simulink model "decimation"  (R2013b)
settings: Solver=ode45  StartTime=0.0  StopTime=10.0  RelTol=1e-3
undefined symbols (not defined in the file): xlfda_numerator
libraries: xbsIndex_r4 x1962, xps_library x2, casper_library_misc x1
(part 1 of 19)
settings Model: Creator=root  LastModifiedBy=root

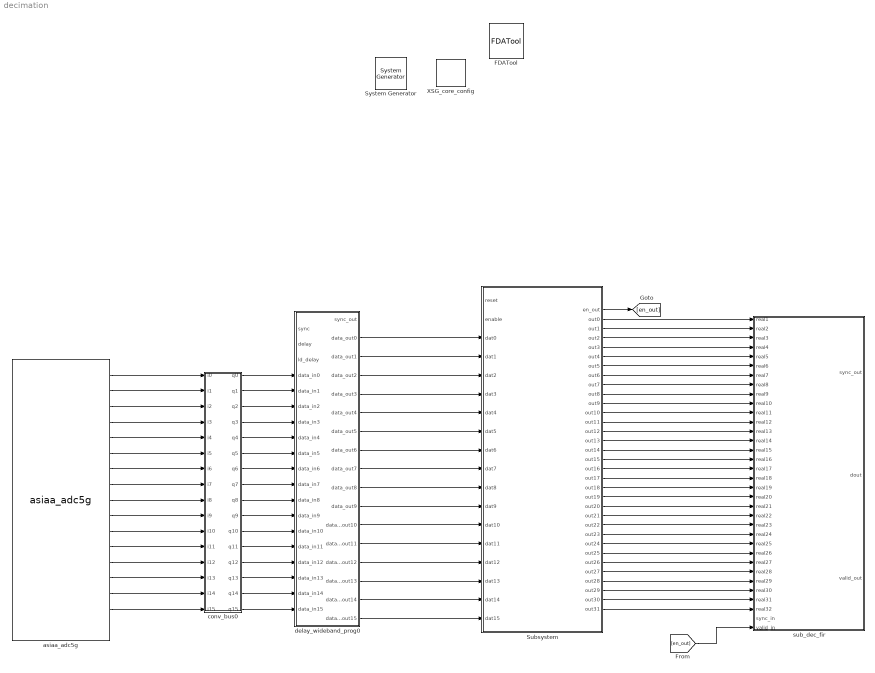
== system decimation ==
  " System Generator" : xbsIndex_r4/ System Generator  Tag=genX  xilinxfamily=Kintex7  part=xc7k325t  speed=-3  package=fbg676  synthesis_tool=XST  clock_wrapper=Clock Enables  directory=./netlist  proj_type=Project Navigator  Synth_file=XST Defaults  Impl_file=ISE Defaults  testbench=off  simulink_period=1  sysclk_period=10  dcm_input_clock_period=10  incr_netlist=off  trim_vbits=Everywhere in SubSystem  dbl_ovrd=According to Block Masks  core_generation=According to Block Masks  run_coregen=off  deprecated_control=off  eval_field=0  block_type=sysgen
  FDATool : xbsIndex_r4/FDATool  block_type=fdatool
      settings: infoedit=FDATool
  Subsystem : Subsystem
  XSG_core_config : xps_library/XSG_core_config  Tag=xps:xsg  hw_sys=ROACH2:sx475t  clk_src=sys_clk  ROACH_clk_src=sys_clk  ROACH2_clk_src=sys_clk  MKDIG_clk_src=sys_clk  clk_rate=100  sample_period=1  synthesis_tool=XST
  asiaa_adc5g : xps_library/ADCs/asiaa_adc5g  Tag=xps:adc5g  input_mode=One-channel -- A  adc_brd=ZDOK 0  demux=1:2  adc_bit_width=4  adc_clk_rate=2500  using_ctrl=on  test_ramp=off
  conv_bus0 : Subsystem
  delay_wideband_prog0 : Subsystem  AncestorBlock=casper_library_delays/delay_wideband_prog  mask(delay_wideband_prog){max_delay=64, n_inputs_bits=4, bram_latency=2, bram_type=Dual Port, async=off}
      mask prompts: max_delay "Max Delay (Sample Clks)"; n_inputs_bits "Number of Simultaneous Inputs(2^?)"; bram_latency "BRAM Latency"; bram_type "Select type of BRAM"; async "asynchronous operation"
      mask init:
      | delay_wideband_prog_init(gcb,...
      |     'max_delay',max_delay,...
      |     'n_inputs_bits',n_inputs_bits,...
      |     'bram_latency',bram_latency,...
      |     'bram_type',bram_type, ...
      |     'async', async);
      mask TypeOptions bram_type: Single Port | Dual Port
  sub_dec_fir : Subsystem
  wires:
  asiaa_adc5g/1 -> conv_bus0/1(i0)
  asiaa_adc5g/2 -> conv_bus0/2(i1)
  asiaa_adc5g/3 -> conv_bus0/3(i2)
  asiaa_adc5g/4 -> conv_bus0/4(i3)
  asiaa_adc5g/5 -> conv_bus0/5(i4)
  asiaa_adc5g/6 -> conv_bus0/6(i5)
  asiaa_adc5g/7 -> conv_bus0/7(i6)
  asiaa_adc5g/8 -> conv_bus0/8(i7)
  asiaa_adc5g/9 -> conv_bus0/9(i8)
  asiaa_adc5g/10 -> conv_bus0/10(i9)
  asiaa_adc5g/11 -> conv_bus0/11(i10)
  asiaa_adc5g/12 -> conv_bus0/12(i11)
  asiaa_adc5g/13 -> conv_bus0/13(i12)
  asiaa_adc5g/14 -> conv_bus0/14(i13)
  asiaa_adc5g/15 -> conv_bus0/15(i14)
  asiaa_adc5g/16 -> conv_bus0/16(i15)
  conv_bus0/1(q0) -> delay_wideband_prog0/4(data_in0)
  conv_bus0/2(q1) -> delay_wideband_prog0/5(data_in1)
  conv_bus0/3(q2) -> delay_wideband_prog0/6(data_in2)
  conv_bus0/4(q3) -> delay_wideband_prog0/7(data_in3)
  conv_bus0/5(q4) -> delay_wideband_prog0/8(data_in4)
  conv_bus0/6(q5) -> delay_wideband_prog0/9(data_in5)
  conv_bus0/7(q6) -> delay_wideband_prog0/10(data_in6)
  conv_bus0/8(q7) -> delay_wideband_prog0/11(data_in7)
  conv_bus0/9(q8) -> delay_wideband_prog0/12(data_in8)
  conv_bus0/10(q9) -> delay_wideband_prog0/13(data_in9)
  conv_bus0/11(q10) -> delay_wideband_prog0/14(data_in10)
  conv_bus0/12(q11) -> delay_wideband_prog0/15(data_in11)
  conv_bus0/13(q12) -> delay_wideband_prog0/16(data_in12)
  conv_bus0/14(q13) -> delay_wideband_prog0/17(data_in13)
  conv_bus0/15(q14) -> delay_wideband_prog0/18(data_in14)
  conv_bus0/16(q15) -> delay_wideband_prog0/19(data_in15)
  delay_wideband_prog0/2(data_out0) -> Subsystem/3(dat0)
  delay_wideband_prog0/3(data_out1) -> Subsystem/4(dat1)
  delay_wideband_prog0/4(data_out2) -> Subsystem/5(dat2)
  delay_wideband_prog0/5(data_out3) -> Subsystem/6(dat3)
  delay_wideband_prog0/6(data_out4) -> Subsystem/7(dat4)
  delay_wideband_prog0/7(data_out5) -> Subsystem/8(dat5)
  delay_wideband_prog0/8(data_out6) -> Subsystem/9(dat6)
  delay_wideband_prog0/9(data_out7) -> Subsystem/10(dat7)
  delay_wideband_prog0/10(data_out8) -> Subsystem/11(dat8)
  delay_wideband_prog0/11(data_out9) -> Subsystem/12(dat9)
  delay_wideband_prog0/12(data_out10) -> Subsystem/13(dat10)
  delay_wideband_prog0/13(data_out11) -> Subsystem/14(dat11)
  delay_wideband_prog0/14(data_out12) -> Subsystem/15(dat12)
  delay_wideband_prog0/15(data_out13) -> Subsystem/16(dat13)
  delay_wideband_prog0/16(data_out14) -> Subsystem/17(dat14)
  delay_wideband_prog0/17(data_out15) -> Subsystem/18(dat15)
  Subsystem/2(out0) -> sub_dec_fir/1(real1)
  Subsystem/3(out1) -> sub_dec_fir/2(real2)
  Subsystem/4(out2) -> sub_dec_fir/3(real3)
  Subsystem/5(out3) -> sub_dec_fir/4(real4)
  Subsystem/6(out4) -> sub_dec_fir/5(real5)
  Subsystem/7(out5) -> sub_dec_fir/6(real6)
  Subsystem/8(out6) -> sub_dec_fir/7(real7)
  Subsystem/9(out7) -> sub_dec_fir/8(real8)
  Subsystem/10(out8) -> sub_dec_fir/9(real9)
  Subsystem/11(out9) -> sub_dec_fir/10(real10)
  Subsystem/12(out10) -> sub_dec_fir/11(real11)
  Subsystem/13(out11) -> sub_dec_fir/12(real12)
  Subsystem/14(out12) -> sub_dec_fir/13(real13)
  Subsystem/15(out13) -> sub_dec_fir/14(real14)
  Subsystem/16(out14) -> sub_dec_fir/15(real15)
  Subsystem/17(out15) -> sub_dec_fir/16(real16)
  Subsystem/18(out16) -> sub_dec_fir/17(real17)
  Subsystem/19(out17) -> sub_dec_fir/18(real18)
  Subsystem/20(out18) -> sub_dec_fir/19(real19)
  Subsystem/21(out19) -> sub_dec_fir/20(real20)
  Subsystem/22(out20) -> sub_dec_fir/21(real21)
  Subsystem/23(out21) -> sub_dec_fir/22(real22)
  Subsystem/24(out22) -> sub_dec_fir/23(real23)
  Subsystem/25(out23) -> sub_dec_fir/24(real24)
  Subsystem/26(out24) -> sub_dec_fir/25(real25)
  Subsystem/27(out25) -> sub_dec_fir/26(real26)
  Subsystem/28(out26) -> sub_dec_fir/27(real27)
  Subsystem/29(out27) -> sub_dec_fir/28(real28)
  Subsystem/30(out28) -> sub_dec_fir/29(real29)
  Subsystem/31(out29) -> sub_dec_fir/30(real30)
  Subsystem/32(out30) -> sub_dec_fir/31(real31)
  Subsystem/33(out31) -> sub_dec_fir/32(real32)
  Subsystem/1(en_out) -> [en_out]
  [en_out] -> sub_dec_fir/34(valid_in)

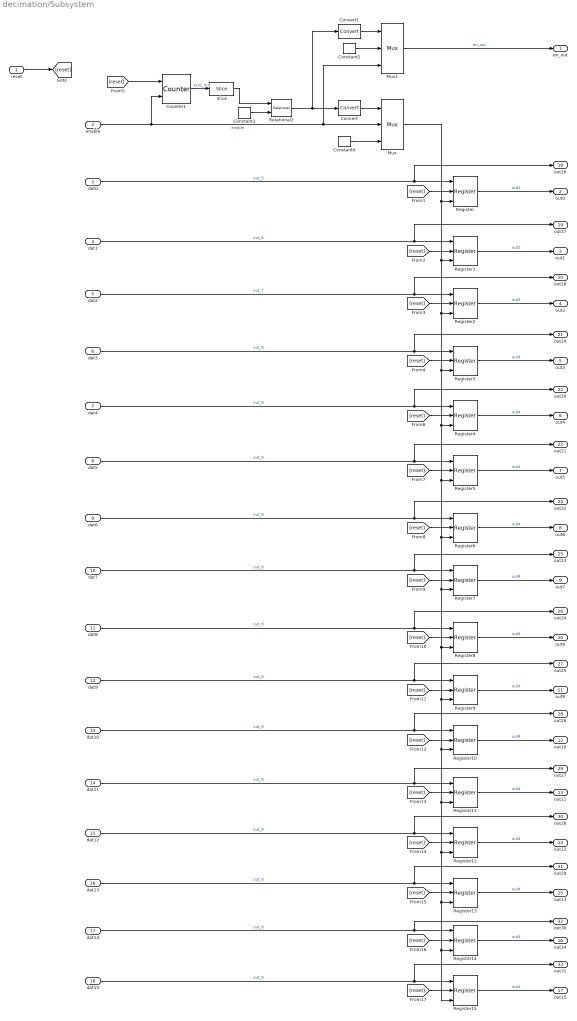
== system decimation/Subsystem ==
  reset : Inport
  enable : Inport  Port=2
  dat0 : Inport  Port=3
  dat1 : Inport  Port=4
  dat2 : Inport  Port=5
  dat3 : Inport  Port=6
  dat4 : Inport  Port=7
  dat5 : Inport  Port=8
  dat6 : Inport  Port=9
  dat7 : Inport  Port=10
  dat8 : Inport  Port=11
  dat9 : Inport  Port=12
  dat10 : Inport  Port=13
  dat11 : Inport  Port=14
  dat12 : Inport  Port=15
  dat13 : Inport  Port=16
  dat14 : Inport  Port=17
  dat15 : Inport  Port=18
  Constant2 : xbsIndex_r4/Constant  const=0  gui_display_data_type=Boolean  arith_type=Boolean  n_bits=2  bin_pt=0  preci_type=Single  exp_width=8  frac_width=24  explicit_period=on  period=1  equ=P=C  opselect=C  inp2=PCIN>>17  opr=+  inp1=P  carry=CIN  dbl_ovrd=off  block_type=constant
  Constant3 : xbsIndex_r4/Constant  const=1  gui_display_data_type=Fixed-point  arith_type=Unsigned  n_bits=2  bin_pt=0  preci_type=Single  exp_width=8  frac_width=24  explicit_period=on  period=1  equ=P=C  opselect=C  inp2=PCIN>>17  opr=+  inp1=P  carry=CIN  dbl_ovrd=off  block_type=constant
  Constant4 : xbsIndex_r4/Constant  const=0  gui_display_data_type=Boolean  arith_type=Boolean  n_bits=2  bin_pt=0  preci_type=Single  exp_width=8  frac_width=24  explicit_period=on  period=1  equ=P=C  opselect=C  inp2=PCIN>>17  opr=+  inp1=P  carry=CIN  dbl_ovrd=off  block_type=constant
  Convert : xbsIndex_r4/Convert  gui_display_data_type=Fixed-point  arith_type=Unsigned  n_bits=1  bin_pt=0  float_type=Single  exp_bits=8  fraction_bits=24  quantization=Truncate  overflow=Wrap  en=off  latency=0  dbl_ovrd=off  pipeline=off  block_type=convert
  Convert1 : xbsIndex_r4/Convert  gui_display_data_type=Fixed-point  arith_type=Unsigned  n_bits=1  bin_pt=0  float_type=Single  exp_bits=8  fraction_bits=24  quantization=Truncate  overflow=Wrap  en=off  latency=0  dbl_ovrd=off  pipeline=off  block_type=convert
  Counter1 : xbsIndex_r4/Counter  cnt_type=Free Running  cnt_to=Inf  operation=Up  start_count=0  cnt_by_val=1  arith_type=Unsigned  n_bits=4  bin_pt=0  load_pin=off  rst=on  en=on  explicit_period=on  period=1  dbl_ovrd=off  use_behavioral_HDL=off  implementation=Fabric  block_type=counter
  Mux : xbsIndex_r4/Mux  inputs=2  en=off  latency=0  precision=Full  arith_type=Unsigned  n_bits=16  bin_pt=14  quantization=Truncate  overflow=Wrap  dbl_ovrd=off  block_type=mux
  Mux1 : xbsIndex_r4/Mux  inputs=2  en=off  latency=0  precision=Full  arith_type=Unsigned  n_bits=16  bin_pt=14  quantization=Truncate  overflow=Wrap  dbl_ovrd=off  block_type=mux
  Register{,1..15} (16 alike) : xbsIndex_r4/Register  init=0  rst=on  en=on  dbl_ovrd=off  block_type=register
  Relational2 : xbsIndex_r4/Relational  mode=a=b  en=off  latency=0  dbl_ovrd=off  block_type=relational
  Slice : xbsIndex_r4/Slice  nbits=1  boolean_output=off  mode=Lower Bit Location + Width  bit1=0  base1=MSB of Input  bit0=0  base0=LSB of Input  dbl_ovrd=off  block_type=slice
  en_out : Outport
  out0 : Outport  Port=2
  out1 : Outport  Port=3
  out2 : Outport  Port=4
  out3 : Outport  Port=5
  out4 : Outport  Port=6
  out5 : Outport  Port=7
  out6 : Outport  Port=8
  out7 : Outport  Port=9
  out8 : Outport  Port=10
  out9 : Outport  Port=11
  out10 : Outport  Port=12
  out11 : Outport  Port=13
  out12 : Outport  Port=14
  out13 : Outport  Port=15
  out14 : Outport  Port=16
  out15 : Outport  Port=17
  out16 : Outport  Port=18
  out17 : Outport  Port=19
  out18 : Outport  Port=20
  out19 : Outport  Port=21
  out20 : Outport  Port=22
  out21 : Outport  Port=23
  out22 : Outport  Port=24
  out23 : Outport  Port=25
  out24 : Outport  Port=26
  out25 : Outport  Port=27
  out26 : Outport  Port=28
  out27 : Outport  Port=29
  out28 : Outport  Port=30
  out29 : Outport  Port=31
  out30 : Outport  Port=32
  out31 : Outport  Port=33
  wires:
  reset/1 -> [reset]
  [reset] -> Register/2
  enable/1 -> Counter1/2, Mux1/3, Mux/2  "enable"
  dat0/1 -> out16/1, Register/1  "out_5"
  [reset] -> Register1/2
  dat1/1 -> out17/1, Register1/1  "out_6"
  Register/1 -> out0/1  "out1"
  [reset] -> Register2/2
  dat2/1 -> out18/1, Register2/1  "out_7"
  [reset] -> Register3/2
  dat3/1 -> out19/1, Register3/1  "out_8"
  Counter1/1 -> Slice/1  "sync_out"
  [reset] -> Counter1/1
  Register1/1 -> out1/1  "out2"
  Register2/1 -> out2/1  "out3"
  Register3/1 -> out3/1  "out4"
  Convert/1 -> Mux/1
  Constant3/1 -> Relational2/2
  Relational2/1 -> Convert1/1, Convert/1
  Constant4/1 -> Mux/3
  Slice/1 -> Relational2/1
  Convert1/1 -> Mux1/1
  Constant2/1 -> Mux1/2
  Mux1/1 -> en_out/1  "en_out"
  [reset] -> Register4/2
  dat4/1 -> out20/1, Register4/1  "out_8"
  Register4/1 -> out4/1  "out4"
  [reset] -> Register5/2
  dat5/1 -> out21/1, Register5/1  "out_8"
  Register5/1 -> out5/1  "out4"
  [reset] -> Register6/2
  dat6/1 -> out22/1, Register6/1  "out_8"
  Register6/1 -> out6/1  "out4"
  [reset] -> Register7/2
  dat7/1 -> out23/1, Register7/1  "out_8"
  Register7/1 -> out7/1  "out4"
  [reset] -> Register8/2
  dat8/1 -> out24/1, Register8/1  "out_8"
  Register8/1 -> out8/1  "out4"
  [reset] -> Register9/2
  dat9/1 -> out25/1, Register9/1  "out_8"
  Register9/1 -> out9/1  "out4"
  [reset] -> Register10/2
  dat10/1 -> out26/1, Register10/1  "out_8"
  Register10/1 -> out10/1  "out4"
  [reset] -> Register11/2
  dat11/1 -> out27/1, Register11/1  "out_8"
  Register11/1 -> out11/1  "out4"
  [reset] -> Register12/2
  dat12/1 -> out28/1, Register12/1  "out_8"
  Register12/1 -> out12/1  "out4"
  [reset] -> Register13/2
  dat13/1 -> out29/1, Register13/1  "out_8"
  Register13/1 -> out13/1  "out4"
  [reset] -> Register14/2
  dat14/1 -> out30/1, Register14/1  "out_8"
  Register14/1 -> out14/1  "out4"
  Mux/1 -> Register/3, Register1/3, Register2/3, Register10/3, Register13/3, Register15/3, Register14/3, Register12/3, Register11/3, Register9/3, Register8/3, Register7/3, Register6/3, Register5/3, Register4/3, Register3/3
  [reset] -> Register15/2
  dat15/1 -> out31/1, Register15/1  "out_8"
  Register15/1 -> out15/1  "out4"

== system decimation/conv_bus0 ==
  i0 : Inport
  i1 : Inport  Port=2
  i2 : Inport  Port=3
  i3 : Inport  Port=4
  i4 : Inport  Port=5
  i5 : Inport  Port=6
  i6 : Inport  Port=7
  i7 : Inport  Port=8
  i8 : Inport  Port=9
  i9 : Inport  Port=10
  i10 : Inport  Port=11
  i11 : Inport  Port=12
  i12 : Inport  Port=13
  i13 : Inport  Port=14
  i14 : Inport  Port=15
  i15 : Inport  Port=16
  conv_ob0 : Subsystem
  conv_ob1 : Subsystem
  conv_ob10 : Subsystem
  conv_ob11 : Subsystem
  conv_ob12 : Subsystem
  conv_ob13 : Subsystem
  conv_ob14 : Subsystem
  conv_ob15 : Subsystem
  conv_ob2 : Subsystem
  conv_ob3 : Subsystem
  conv_ob4 : Subsystem
  conv_ob5 : Subsystem
  conv_ob6 : Subsystem
  conv_ob7 : Subsystem
  conv_ob8 : Subsystem
  conv_ob9 : Subsystem
  q0 : Outport
  q1 : Outport  Port=2
  q2 : Outport  Port=3
  q3 : Outport  Port=4
  q4 : Outport  Port=5
  q5 : Outport  Port=6
  q6 : Outport  Port=7
  q7 : Outport  Port=8
  q8 : Outport  Port=9
  q9 : Outport  Port=10
  q10 : Outport  Port=11
  q11 : Outport  Port=12
  q12 : Outport  Port=13
  q13 : Outport  Port=14
  q14 : Outport  Port=15
  q15 : Outport  Port=16
  wires:
  conv_ob7/1(q) -> q7/1
  i7/1 -> conv_ob7/1(i)
  conv_ob6/1(q) -> q6/1
  i6/1 -> conv_ob6/1(i)
  conv_ob5/1(q) -> q5/1
  i5/1 -> conv_ob5/1(i)
  conv_ob4/1(q) -> q4/1
  i4/1 -> conv_ob4/1(i)
  conv_ob3/1(q) -> q3/1
  i3/1 -> conv_ob3/1(i)
  conv_ob2/1(q) -> q2/1
  i2/1 -> conv_ob2/1(i)
  conv_ob1/1(q) -> q1/1
  i1/1 -> conv_ob1/1(i)
  conv_ob0/1(q) -> q0/1
  i0/1 -> conv_ob0/1(i)
  conv_ob15/1(q) -> q15/1
  i15/1 -> conv_ob15/1(i)
  conv_ob14/1(q) -> q14/1
  i14/1 -> conv_ob14/1(i)
  conv_ob13/1(q) -> q13/1
  i13/1 -> conv_ob13/1(i)
  conv_ob12/1(q) -> q12/1
  i12/1 -> conv_ob12/1(i)
  conv_ob11/1(q) -> q11/1
  i11/1 -> conv_ob11/1(i)
  conv_ob10/1(q) -> q10/1
  i10/1 -> conv_ob10/1(i)
  conv_ob9/1(q) -> q9/1
  i9/1 -> conv_ob9/1(i)
  conv_ob8/1(q) -> q8/1
  i8/1 -> conv_ob8/1(i)

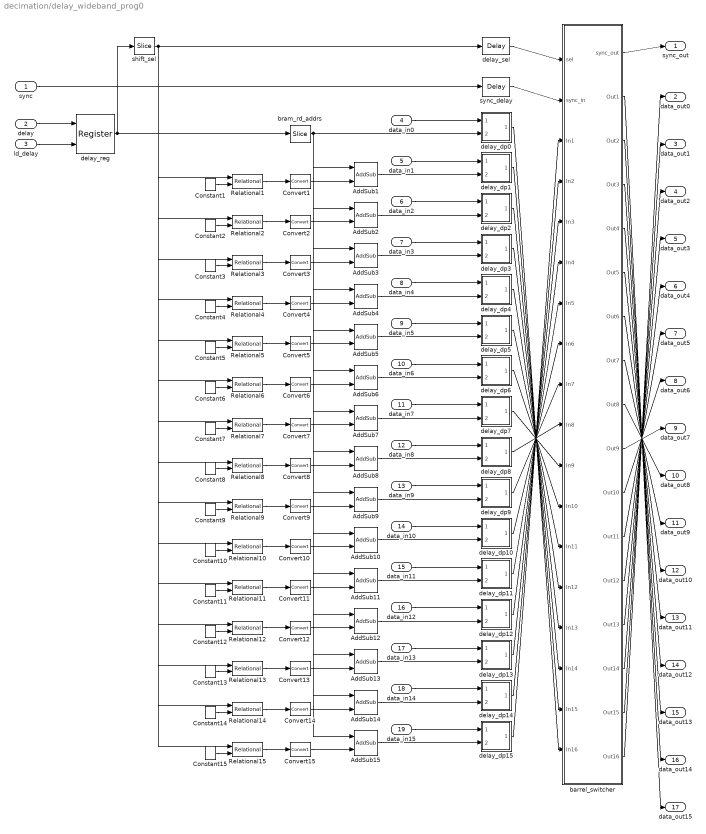
== system decimation/delay_wideband_prog0 ==
  sync : Inport
  delay : Inport  Port=2
  ld_delay : Inport  Port=3
  data_in0 : Inport  Port=4
  data_in1 : Inport  Port=5
  data_in2 : Inport  Port=6
  data_in3 : Inport  Port=7
  data_in4 : Inport  Port=8
  data_in5 : Inport  Port=9
  data_in6 : Inport  Port=10
  data_in7 : Inport  Port=11
  data_in8 : Inport  Port=12
  data_in9 : Inport  Port=13
  data_in10 : Inport  Port=14
  data_in11 : Inport  Port=15
  data_in12 : Inport  Port=16
  data_in13 : Inport  Port=17
  data_in14 : Inport  Port=18
  data_in15 : Inport  Port=19
  AddSub{1..15} (15 alike) : xbsIndex_r4/AddSub  mode=Addition  use_carryin=off  use_carryout=off  en=off  latency=0  precision=Full  arith_type=Unsigned  n_bits=2  bin_pt=0  quantization=Truncate  overflow=Wrap  dbl_ovrd=off  use_behavioral_HDL=off  hw_selection=Fabric  pipelined=off  block_type=addsub
  Constant1 : xbsIndex_r4/Constant  const=14  gui_display_data_type=Fixed-point  arith_type=Unsigned  n_bits=4  bin_pt=0  preci_type=Single  exp_width=8  frac_width=24  explicit_period=on  period=1  equ=P=C  opselect=C  inp2=PCIN>>17  opr=+  inp1=P  carry=CIN  dbl_ovrd=off  block_type=constant
  Constant10 : xbsIndex_r4/Constant  const=5  gui_display_data_type=Fixed-point  arith_type=Unsigned  n_bits=4  bin_pt=0  preci_type=Single  exp_width=8  frac_width=24  explicit_period=on  period=1  equ=P=C  opselect=C  inp2=PCIN>>17  opr=+  inp1=P  carry=CIN  dbl_ovrd=off  block_type=constant
  Constant11 : xbsIndex_r4/Constant  const=4  gui_display_data_type=Fixed-point  arith_type=Unsigned  n_bits=4  bin_pt=0  preci_type=Single  exp_width=8  frac_width=24  explicit_period=on  period=1  equ=P=C  opselect=C  inp2=PCIN>>17  opr=+  inp1=P  carry=CIN  dbl_ovrd=off  block_type=constant
  Constant12 : xbsIndex_r4/Constant  const=3  gui_display_data_type=Fixed-point  arith_type=Unsigned  n_bits=4  bin_pt=0  preci_type=Single  exp_width=8  frac_width=24  explicit_period=on  period=1  equ=P=C  opselect=C  inp2=PCIN>>17  opr=+  inp1=P  carry=CIN  dbl_ovrd=off  block_type=constant
  Constant13 : xbsIndex_r4/Constant  const=2  gui_display_data_type=Fixed-point  arith_type=Unsigned  n_bits=4  bin_pt=0  preci_type=Single  exp_width=8  frac_width=24  explicit_period=on  period=1  equ=P=C  opselect=C  inp2=PCIN>>17  opr=+  inp1=P  carry=CIN  dbl_ovrd=off  block_type=constant
  Constant14 : xbsIndex_r4/Constant  const=1  gui_display_data_type=Fixed-point  arith_type=Unsigned  n_bits=4  bin_pt=0  preci_type=Single  exp_width=8  frac_width=24  explicit_period=on  period=1  equ=P=C  opselect=C  inp2=PCIN>>17  opr=+  inp1=P  carry=CIN  dbl_ovrd=off  block_type=constant
  Constant15 : xbsIndex_r4/Constant  const=0  gui_display_data_type=Fixed-point  arith_type=Unsigned  n_bits=4  bin_pt=0  preci_type=Single  exp_width=8  frac_width=24  explicit_period=on  period=1  equ=P=C  opselect=C  inp2=PCIN>>17  opr=+  inp1=P  carry=CIN  dbl_ovrd=off  block_type=constant
  Constant2 : xbsIndex_r4/Constant  const=13  gui_display_data_type=Fixed-point  arith_type=Unsigned  n_bits=4  bin_pt=0  preci_type=Single  exp_width=8  frac_width=24  explicit_period=on  period=1  equ=P=C  opselect=C  inp2=PCIN>>17  opr=+  inp1=P  carry=CIN  dbl_ovrd=off  block_type=constant
  Constant3 : xbsIndex_r4/Constant  const=12  gui_display_data_type=Fixed-point  arith_type=Unsigned  n_bits=4  bin_pt=0  preci_type=Single  exp_width=8  frac_width=24  explicit_period=on  period=1  equ=P=C  opselect=C  inp2=PCIN>>17  opr=+  inp1=P  carry=CIN  dbl_ovrd=off  block_type=constant
  Constant4 : xbsIndex_r4/Constant  const=11  gui_display_data_type=Fixed-point  arith_type=Unsigned  n_bits=4  bin_pt=0  preci_type=Single  exp_width=8  frac_width=24  explicit_period=on  period=1  equ=P=C  opselect=C  inp2=PCIN>>17  opr=+  inp1=P  carry=CIN  dbl_ovrd=off  block_type=constant
  Constant5 : xbsIndex_r4/Constant  const=10  gui_display_data_type=Fixed-point  arith_type=Unsigned  n_bits=4  bin_pt=0  preci_type=Single  exp_width=8  frac_width=24  explicit_period=on  period=1  equ=P=C  opselect=C  inp2=PCIN>>17  opr=+  inp1=P  carry=CIN  dbl_ovrd=off  block_type=constant
  Constant6 : xbsIndex_r4/Constant  const=9  gui_display_data_type=Fixed-point  arith_type=Unsigned  n_bits=4  bin_pt=0  preci_type=Single  exp_width=8  frac_width=24  explicit_period=on  period=1  equ=P=C  opselect=C  inp2=PCIN>>17  opr=+  inp1=P  carry=CIN  dbl_ovrd=off  block_type=constant
  Constant7 : xbsIndex_r4/Constant  const=8  gui_display_data_type=Fixed-point  arith_type=Unsigned  n_bits=4  bin_pt=0  preci_type=Single  exp_width=8  frac_width=24  explicit_period=on  period=1  equ=P=C  opselect=C  inp2=PCIN>>17  opr=+  inp1=P  carry=CIN  dbl_ovrd=off  block_type=constant
  Constant8 : xbsIndex_r4/Constant  const=7  gui_display_data_type=Fixed-point  arith_type=Unsigned  n_bits=4  bin_pt=0  preci_type=Single  exp_width=8  frac_width=24  explicit_period=on  period=1  equ=P=C  opselect=C  inp2=PCIN>>17  opr=+  inp1=P  carry=CIN  dbl_ovrd=off  block_type=constant
  Constant9 : xbsIndex_r4/Constant  const=6  gui_display_data_type=Fixed-point  arith_type=Unsigned  n_bits=4  bin_pt=0  preci_type=Single  exp_width=8  frac_width=24  explicit_period=on  period=1  equ=P=C  opselect=C  inp2=PCIN>>17  opr=+  inp1=P  carry=CIN  dbl_ovrd=off  block_type=constant
  Convert{1..15} (15 alike) : xbsIndex_r4/Convert  gui_display_data_type=Fixed-point  arith_type=Unsigned  n_bits=1  bin_pt=0  float_type=Single  exp_bits=8  fraction_bits=24  quantization=Truncate  overflow=Wrap  en=off  latency=0  dbl_ovrd=off  pipeline=off  block_type=convert
  Relational{1..15} (15 alike) : xbsIndex_r4/Relational  mode=a>b  en=off  latency=0  dbl_ovrd=off  block_type=relational
  barrel_switcher : Subsystem  AncestorBlock=casper_library_reorder/barrel_switcher  mask(barrel_switcher){n_inputs=4, async=off}
      mask prompts: n_inputs "Number of Inputs: (2^?)"; async "Asynchronous operation"
      mask help:
      | Shifts input to right by amount specified on sel,
      | wrapping around into higher order bits.
      mask init:
      | barrel_switcher_init(gcb,...
      |     'n_inputs', n_inputs, ...
      |     'async', async);
      mask Help: eval('xlWeb(''http://casper.berkeley.edu/wiki/Barrel_switcher'')')
  bram_rd_addrs : xbsIndex_r4/Slice  nbits=2  boolean_output=off  mode=Lower Bit Location + Width  bit1=0  base1=MSB of Input  bit0=4  base0=LSB of Input  dbl_ovrd=off  block_type=slice
  delay_dp0 : Subsystem  AncestorBlock=casper_library_delays/delay_bram_prog_dp  mask(delay_bram_prog_dp){ram_bits=2, bram_latency=2, async=off}
      mask prompts: ram_bits "Max delay (2^?)"; bram_latency "BRAM latency"; async "asynchronous operation"
      mask init:
      | delay_bram_prog_dp_init(gcb, ...
      |     'ram_bits', ram_bits, ...
      |     'bram_latency', bram_latency, ...
      |     'async', async);
  delay_dp1 : Subsystem  AncestorBlock=casper_library_delays/delay_bram_prog_dp  mask(delay_bram_prog_dp){ram_bits=2, bram_latency=2, async=off}
      mask prompts: ram_bits "Max delay (2^?)"; bram_latency "BRAM latency"; async "asynchronous operation"
      mask init:
      | delay_bram_prog_dp_init(gcb, ...
      |     'ram_bits', ram_bits, ...
      |     'bram_latency', bram_latency, ...
      |     'async', async);
  delay_dp10 : Subsystem  AncestorBlock=casper_library_delays/delay_bram_prog_dp  mask(delay_bram_prog_dp){ram_bits=2, bram_latency=2, async=off}
      mask prompts: ram_bits "Max delay (2^?)"; bram_latency "BRAM latency"; async "asynchronous operation"
      mask init:
      | delay_bram_prog_dp_init(gcb, ...
      |     'ram_bits', ram_bits, ...
      |     'bram_latency', bram_latency, ...
      |     'async', async);
  delay_dp11 : Subsystem  AncestorBlock=casper_library_delays/delay_bram_prog_dp  mask(delay_bram_prog_dp){ram_bits=2, bram_latency=2, async=off}
      mask prompts: ram_bits "Max delay (2^?)"; bram_latency "BRAM latency"; async "asynchronous operation"
      mask init:
      | delay_bram_prog_dp_init(gcb, ...
      |     'ram_bits', ram_bits, ...
      |     'bram_latency', bram_latency, ...
      |     'async', async);
  delay_dp12 : Subsystem  AncestorBlock=casper_library_delays/delay_bram_prog_dp  mask(delay_bram_prog_dp){ram_bits=2, bram_latency=2, async=off}
      mask prompts: ram_bits "Max delay (2^?)"; bram_latency "BRAM latency"; async "asynchronous operation"
      mask init:
      | delay_bram_prog_dp_init(gcb, ...
      |     'ram_bits', ram_bits, ...
      |     'bram_latency', bram_latency, ...
      |     'async', async);
  delay_dp13 : Subsystem  AncestorBlock=casper_library_delays/delay_bram_prog_dp  mask(delay_bram_prog_dp){ram_bits=2, bram_latency=2, async=off}
      mask prompts: ram_bits "Max delay (2^?)"; bram_latency "BRAM latency"; async "asynchronous operation"
      mask init:
      | delay_bram_prog_dp_init(gcb, ...
      |     'ram_bits', ram_bits, ...
      |     'bram_latency', bram_latency, ...
      |     'async', async);
  delay_dp14 : Subsystem  AncestorBlock=casper_library_delays/delay_bram_prog_dp  mask(delay_bram_prog_dp){ram_bits=2, bram_latency=2, async=off}
      mask prompts: ram_bits "Max delay (2^?)"; bram_latency "BRAM latency"; async "asynchronous operation"
      mask init:
      | delay_bram_prog_dp_init(gcb, ...
      |     'ram_bits', ram_bits, ...
      |     'bram_latency', bram_latency, ...
      |     'async', async);
  delay_dp15 : Subsystem  AncestorBlock=casper_library_delays/delay_bram_prog_dp  mask(delay_bram_prog_dp){ram_bits=2, bram_latency=2, async=off}
      mask prompts: ram_bits "Max delay (2^?)"; bram_latency "BRAM latency"; async "asynchronous operation"
      mask init:
      | delay_bram_prog_dp_init(gcb, ...
      |     'ram_bits', ram_bits, ...
      |     'bram_latency', bram_latency, ...
      |     'async', async);
  delay_dp2 : Subsystem  AncestorBlock=casper_library_delays/delay_bram_prog_dp  mask(delay_bram_prog_dp){ram_bits=2, bram_latency=2, async=off}
      mask prompts: ram_bits "Max delay (2^?)"; bram_latency "BRAM latency"; async "asynchronous operation"
      mask init:
      | delay_bram_prog_dp_init(gcb, ...
      |     'ram_bits', ram_bits, ...
      |     'bram_latency', bram_latency, ...
      |     'async', async);
  delay_dp3 : Subsystem  AncestorBlock=casper_library_delays/delay_bram_prog_dp  mask(delay_bram_prog_dp){ram_bits=2, bram_latency=2, async=off}
      mask prompts: ram_bits "Max delay (2^?)"; bram_latency "BRAM latency"; async "asynchronous operation"
      mask init:
      | delay_bram_prog_dp_init(gcb, ...
      |     'ram_bits', ram_bits, ...
      |     'bram_latency', bram_latency, ...
      |     'async', async);
  delay_dp4 : Subsystem  AncestorBlock=casper_library_delays/delay_bram_prog_dp  mask(delay_bram_prog_dp){ram_bits=2, bram_latency=2, async=off}
      mask prompts: ram_bits "Max delay (2^?)"; bram_latency "BRAM latency"; async "asynchronous operation"
      mask init:
      | delay_bram_prog_dp_init(gcb, ...
      |     'ram_bits', ram_bits, ...
      |     'bram_latency', bram_latency, ...
      |     'async', async);
  delay_dp5 : Subsystem  AncestorBlock=casper_library_delays/delay_bram_prog_dp  mask(delay_bram_prog_dp){ram_bits=2, bram_latency=2, async=off}
      mask prompts: ram_bits "Max delay (2^?)"; bram_latency "BRAM latency"; async "asynchronous operation"
      mask init:
      | delay_bram_prog_dp_init(gcb, ...
      |     'ram_bits', ram_bits, ...
      |     'bram_latency', bram_latency, ...
      |     'async', async);
  delay_dp6 : Subsystem  AncestorBlock=casper_library_delays/delay_bram_prog_dp  mask(delay_bram_prog_dp){ram_bits=2, bram_latency=2, async=off}
      mask prompts: ram_bits "Max delay (2^?)"; bram_latency "BRAM latency"; async "asynchronous operation"
      mask init:
      | delay_bram_prog_dp_init(gcb, ...
      |     'ram_bits', ram_bits, ...
      |     'bram_latency', bram_latency, ...
      |     'async', async);
  delay_dp7 : Subsystem  AncestorBlock=casper_library_delays/delay_bram_prog_dp  mask(delay_bram_prog_dp){ram_bits=2, bram_latency=2, async=off}
      mask prompts: ram_bits "Max delay (2^?)"; bram_latency "BRAM latency"; async "asynchronous operation"
      mask init:
      | delay_bram_prog_dp_init(gcb, ...
      |     'ram_bits', ram_bits, ...
      |     'bram_latency', bram_latency, ...
      |     'async', async);
  delay_dp8 : Subsystem  AncestorBlock=casper_library_delays/delay_bram_prog_dp  mask(delay_bram_prog_dp){ram_bits=2, bram_latency=2, async=off}
      mask prompts: ram_bits "Max delay (2^?)"; bram_latency "BRAM latency"; async "asynchronous operation"
      mask init:
      | delay_bram_prog_dp_init(gcb, ...
      |     'ram_bits', ram_bits, ...
      |     'bram_latency', bram_latency, ...
      |     'async', async);
  delay_dp9 : Subsystem  AncestorBlock=casper_library_delays/delay_bram_prog_dp  mask(delay_bram_prog_dp){ram_bits=2, bram_latency=2, async=off}
      mask prompts: ram_bits "Max delay (2^?)"; bram_latency "BRAM latency"; async "asynchronous operation"
      mask init:
      | delay_bram_prog_dp_init(gcb, ...
      |     'ram_bits', ram_bits, ...
      |     'bram_latency', bram_latency, ...
      |     'async', async);
  delay_reg : xbsIndex_r4/Register  init=0  rst=off  en=on  dbl_ovrd=off  block_type=register
  delay_sel : xbsIndex_r4/Delay  rst=off  infoeditControl=Selection of Reset will increase slice count due to use of real FFs and instead of SRLs  en=off  latency=3  dbl_ovrd=off  reg_retiming=on  block_type=delay
  shift_sel : xbsIndex_r4/Slice  nbits=4  boolean_output=off  mode=Lower Bit Location + Width  bit1=0  base1=MSB of Input  bit0=0  base0=LSB of Input  dbl_ovrd=off  block_type=slice
  sync_delay : xbsIndex_r4/Delay  rst=off  infoeditControl=Selection of Reset will increase slice count due to use of real FFs and instead of SRLs  en=off  latency=3  dbl_ovrd=off  reg_retiming=on  block_type=delay
  sync_out : Outport
  data_out0 : Outport  Port=2
  data_out1 : Outport  Port=3
  data_out2 : Outport  Port=4
  data_out3 : Outport  Port=5
  data_out4 : Outport  Port=6
  data_out5 : Outport  Port=7
  data_out6 : Outport  Port=8
  data_out7 : Outport  Port=9
  data_out8 : Outport  Port=10
  data_out9 : Outport  Port=11
  data_out10 : Outport  Port=12
  data_out11 : Outport  Port=13
  data_out12 : Outport  Port=14
  data_out13 : Outport  Port=15
  data_out14 : Outport  Port=16
  data_out15 : Outport  Port=17
  wires:
  sync/1 -> sync_delay/1
  delay/1 -> delay_reg/1
  ld_delay/1 -> delay_reg/2
  delay_reg/1 -> bram_rd_addrs/1, shift_sel/1
  sync_delay/1 -> barrel_switcher/2(sync_in)
  barrel_switcher/1(sync_out) -> sync_out/1
  shift_sel/1 -> delay_sel/1, Relational1/1, Relational2/1, Relational3/1, Relational4/1, Relational5/1, Relational6/1, Relational7/1, Relational8/1, Relational9/1, Relational10/1, Relational11/1, Relational12/1, Relational13/1, Relational14/1, Relational15/1
  delay_sel/1 -> barrel_switcher/1(sel)
  barrel_switcher/17(Out16) -> data_out0/1
  barrel_switcher/16(Out15) -> data_out1/1
  barrel_switcher/15(Out14) -> data_out2/1
  barrel_switcher/14(Out13) -> data_out3/1
  barrel_switcher/13(Out12) -> data_out4/1
  barrel_switcher/12(Out11) -> data_out5/1
  barrel_switcher/11(Out10) -> data_out6/1
  barrel_switcher/10(Out9) -> data_out7/1
  barrel_switcher/9(Out8) -> data_out8/1
  barrel_switcher/8(Out7) -> data_out9/1
  barrel_switcher/7(Out6) -> data_out10/1
  barrel_switcher/6(Out5) -> data_out11/1
  barrel_switcher/5(Out4) -> data_out12/1
  barrel_switcher/4(Out3) -> data_out13/1
  barrel_switcher/3(Out2) -> data_out14/1
  barrel_switcher/2(Out1) -> data_out15/1
  data_in0/1 -> delay_dp0/1(din)
  delay_dp0/1(dout) -> barrel_switcher/18(In16)
  bram_rd_addrs/1 -> delay_dp0/2(delay), AddSub1/1, AddSub2/1, AddSub3/1, AddSub4/1, AddSub5/1, AddSub6/1, AddSub7/1, AddSub8/1, AddSub9/1, AddSub10/1, AddSub11/1, AddSub12/1, AddSub13/1, AddSub14/1, AddSub15/1
  data_in1/1 -> delay_dp1/1(din)
  delay_dp1/1(dout) -> barrel_switcher/17(In15)
  Constant1/1 -> Relational1/2
  Relational1/1 -> Convert1/1
  Convert1/1 -> AddSub1/2
  AddSub1/1 -> delay_dp1/2(delay)
  data_in2/1 -> delay_dp2/1(din)
  delay_dp2/1(dout) -> barrel_switcher/16(In14)
  Constant2/1 -> Relational2/2
  Relational2/1 -> Convert2/1
  Convert2/1 -> AddSub2/2
  AddSub2/1 -> delay_dp2/2(delay)
  data_in3/1 -> delay_dp3/1(din)
  delay_dp3/1(dout) -> barrel_switcher/15(In13)
  Constant3/1 -> Relational3/2
  Relational3/1 -> Convert3/1
  Convert3/1 -> AddSub3/2
  AddSub3/1 -> delay_dp3/2(delay)
  data_in4/1 -> delay_dp4/1(din)
  delay_dp4/1(dout) -> barrel_switcher/14(In12)
  Constant4/1 -> Relational4/2
  Relational4/1 -> Convert4/1
  Convert4/1 -> AddSub4/2
  AddSub4/1 -> delay_dp4/2(delay)
  data_in5/1 -> delay_dp5/1(din)
  delay_dp5/1(dout) -> barrel_switcher/13(In11)
  Constant5/1 -> Relational5/2
  Relational5/1 -> Convert5/1
  Convert5/1 -> AddSub5/2
  AddSub5/1 -> delay_dp5/2(delay)
  data_in6/1 -> delay_dp6/1(din)
  delay_dp6/1(dout) -> barrel_switcher/12(In10)
  Constant6/1 -> Relational6/2
  Relational6/1 -> Convert6/1
  Convert6/1 -> AddSub6/2
  AddSub6/1 -> delay_dp6/2(delay)
  data_in7/1 -> delay_dp7/1(din)
  delay_dp7/1(dout) -> barrel_switcher/11(In9)
  Constant7/1 -> Relational7/2
  Relational7/1 -> Convert7/1
  Convert7/1 -> AddSub7/2
  AddSub7/1 -> delay_dp7/2(delay)
  data_in8/1 -> delay_dp8/1(din)
  delay_dp8/1(dout) -> barrel_switcher/10(In8)
  Constant8/1 -> Relational8/2
  Relational8/1 -> Convert8/1
  Convert8/1 -> AddSub8/2
  AddSub8/1 -> delay_dp8/2(delay)
  data_in9/1 -> delay_dp9/1(din)
  delay_dp9/1(dout) -> barrel_switcher/9(In7)
  Constant9/1 -> Relational9/2
  Relational9/1 -> Convert9/1
  Convert9/1 -> AddSub9/2
  AddSub9/1 -> delay_dp9/2(delay)
  data_in10/1 -> delay_dp10/1(din)
  delay_dp10/1(dout) -> barrel_switcher/8(In6)
  Constant10/1 -> Relational10/2
  Relational10/1 -> Convert10/1
  Convert10/1 -> AddSub10/2
  AddSub10/1 -> delay_dp10/2(delay)
  data_in11/1 -> delay_dp11/1(din)
  delay_dp11/1(dout) -> barrel_switcher/7(In5)
  Constant11/1 -> Relational11/2
  Relational11/1 -> Convert11/1
  Convert11/1 -> AddSub11/2
  AddSub11/1 -> delay_dp11/2(delay)
  data_in12/1 -> delay_dp12/1(din)
  delay_dp12/1(dout) -> barrel_switcher/6(In4)
  Constant12/1 -> Relational12/2
  Relational12/1 -> Convert12/1
  Convert12/1 -> AddSub12/2
  AddSub12/1 -> delay_dp12/2(delay)
  data_in13/1 -> delay_dp13/1(din)
  delay_dp13/1(dout) -> barrel_switcher/5(In3)
  Constant13/1 -> Relational13/2
  Relational13/1 -> Convert13/1
  Convert13/1 -> AddSub13/2
  AddSub13/1 -> delay_dp13/2(delay)
  data_in14/1 -> delay_dp14/1(din)
  delay_dp14/1(dout) -> barrel_switcher/4(In2)
  Constant14/1 -> Relational14/2
  Relational14/1 -> Convert14/1
  Convert14/1 -> AddSub14/2
  AddSub14/1 -> delay_dp14/2(delay)
  data_in15/1 -> delay_dp15/1(din)
  delay_dp15/1(dout) -> barrel_switcher/3(In1)
  Constant15/1 -> Relational15/2
  Relational15/1 -> Convert15/1
  Convert15/1 -> AddSub15/2
  AddSub15/1 -> delay_dp15/2(delay)

== system decimation/sub_dec_fir ==
  real1 : Inport
  real2 : Inport  Port=2
  real3 : Inport  Port=3
  real4 : Inport  Port=4
  real5 : Inport  Port=5
  real6 : Inport  Port=6
  real7 : Inport  Port=7
  real8 : Inport  Port=8
  real9 : Inport  Port=9
  real10 : Inport  Port=10
  real11 : Inport  Port=11
  real12 : Inport  Port=12
  real13 : Inport  Port=13
  real14 : Inport  Port=14
  real15 : Inport  Port=15
  real16 : Inport  Port=16
  real17 : Inport  Port=17
  real18 : Inport  Port=18
  real19 : Inport  Port=19
  real20 : Inport  Port=20
  real21 : Inport  Port=21
  real22 : Inport  Port=22
  real23 : Inport  Port=23
  real24 : Inport  Port=24
  real25 : Inport  Port=25
  real26 : Inport  Port=26
  real27 : Inport  Port=27
  real28 : Inport  Port=28
  real29 : Inport  Port=29
  real30 : Inport  Port=30
  real31 : Inport  Port=31
  real32 : Inport  Port=32
  sync_in : Inport  Port=33
  valid_in : Inport  Port=34
  Constant{1..3,5..12,14..34} (32 alike) : xbsIndex_r4/Constant  const=0  gui_display_data_type=Fixed-point  arith_type=Signed (2's comp)  n_bits=8  bin_pt=7  preci_type=Single  exp_width=8  frac_width=24  explicit_period=on  period=1  equ=P=C  opselect=C  inp2=PCIN>>17  opr=+  inp1=P  carry=CIN  dbl_ovrd=off  block_type=constant
  FDATool : xbsIndex_r4/FDATool  block_type=fdatool
      settings: infoedit=FDATool
  dec_fir_async : Subsystem  Tag=casper:dec_fir_async  AncestorBlock=casper_library_downconverter/dec_fir_async  mask(dec_fir_async){n_inputs=32, coeff=xlfda_numerator('FDATool'), output_width=8, output_bp=7, quantization=Round  (unbiased: +/- Inf), add_latency=1, mult_latency=2, conv_latency=2, coeff_bit_width=25, coeff_bin_pt=24, lshift=1, absorb_adders=on, adder_imp=DSP48, async=on, bus_input=off, input_width=0, input_bp=0, input_type=Signed}
      mask prompts: n_inputs "Number of Parallel Streams"; coeff "Coefficients"; output_width "Output bitwidth"; output_bp "Output binary point"; quantization "Quantization Behavior"; add_latency "Add Latency"; mult_latency "Mult Latency"; conv_latency "Convert latency"; coeff_bit_width "Coefficient bitwidth"; coeff_bin_pt "Coefficient binary point"; lshift "Post adder-tree shift"; absorb_adders "Absorb adders into DSP slices"; adder_imp "Adder implementation"; async "Asynchronous ops"; bus_input "Bus input"; input_width "Input bitwidth"; input_bp "Input binary point"; input_type "Input datatype"
      mask help: FIR filter which can handle multiple time samples in parallel and decimates down to 1 time sample. If coefficients are symmetric, will automatically fold before multiplying.
      mask init:
      | dec_fir_async_init(gcb);
      settings: AttributesFormatString=|
      | 224 taps
      | 8_7 r/i
      mask TypeOptions quantization: Truncate | Round  (unbiased: +/- Inf) | Round  (unbiased: Even Values)
      mask TypeOptions adder_imp: Behavioral | Fabric | DSP48
      mask Callback bus_input:
      | onoff = get_param(gcb, 'bus_input');
      | set_param_state(gcb, 'input_width', onoff)
      | set_param_state(gcb, 'input_bp', onoff)
      | set_param_state(gcb, 'input_type', onoff)
      mask TypeOptions input_type: Signed | Unsigned
  sync_out : Outport
  dout : Outport  Port=2
  valid_out : Outport  Port=3
  wires:
  real9/1 -> dec_fir_async/19(real9)
  Constant2/1 -> dec_fir_async/6(imag2)
  Constant24/1 -> dec_fir_async/46(imag22)
  real20/1 -> dec_fir_async/41(real20)
  real21/1 -> dec_fir_async/43(real21)
  real17/1 -> dec_fir_async/35(real17)
  real13/1 -> dec_fir_async/27(real13)
  Constant14/1 -> dec_fir_async/26(imag12)
  Constant6/1 -> dec_fir_async/12(imag5)
  real6/1 -> dec_fir_async/13(real6)
  real15/1 -> dec_fir_async/31(real15)
  real2/1 -> dec_fir_async/5(real2)
  real10/1 -> dec_fir_async/21(real10)
  real25/1 -> dec_fir_async/51(real25)
  real18/1 -> dec_fir_async/37(real18)
  real28/1 -> dec_fir_async/57(real28)
  real22/1 -> dec_fir_async/45(real22)
  real14/1 -> dec_fir_async/29(real14)
  Constant31/1 -> dec_fir_async/60(imag29)
  real31/1 -> dec_fir_async/63(real31)
  Constant30/1 -> dec_fir_async/58(imag28)
  Constant23/1 -> dec_fir_async/44(imag21)
  real29/1 -> dec_fir_async/59(real29)
  real5/1 -> dec_fir_async/11(real5)
  Constant10/1 -> dec_fir_async/20(imag9)
  Constant7/1 -> dec_fir_async/14(imag6)
  Constant26/1 -> dec_fir_async/50(imag24)
  real7/1 -> dec_fir_async/15(real7)
  Constant32/1 -> dec_fir_async/62(imag30)
  Constant9/1 -> dec_fir_async/18(imag8)
  Constant29/1 -> dec_fir_async/56(imag27)
  real26/1 -> dec_fir_async/53(real26)
  Constant22/1 -> dec_fir_async/42(imag20)
  dec_fir_async/1(sync_out) -> sync_out/1
  real8/1 -> dec_fir_async/17(real8)
  real27/1 -> dec_fir_async/55(real27)
  dec_fir_async/2(dout) -> dout/1
  Constant18/1 -> dec_fir_async/34(imag16)
  Constant25/1 -> dec_fir_async/48(imag23)
  sync_in/1 -> dec_fir_async/1(sync_in)
  Constant21/1 -> dec_fir_async/40(imag19)
  real3/1 -> dec_fir_async/7(real3)
  Constant34/1 -> dec_fir_async/66(imag32)
  real11/1 -> dec_fir_async/23(real11)
  Constant8/1 -> dec_fir_async/16(imag7)
  real19/1 -> dec_fir_async/39(real19)
  Constant17/1 -> dec_fir_async/32(imag15)
  Constant1/1 -> dec_fir_async/4(imag1)
  real12/1 -> dec_fir_async/25(real12)
  Constant20/1 -> dec_fir_async/38(imag18)
  Constant16/1 -> dec_fir_async/30(imag14)
  Constant5/1 -> dec_fir_async/10(imag4)
  Constant15/1 -> dec_fir_async/28(imag13)
  real32/1 -> dec_fir_async/65(real32)
  real30/1 -> dec_fir_async/61(real30)
  Constant19/1 -> dec_fir_async/36(imag17)
  real4/1 -> dec_fir_async/9(real4)
  Constant11/1 -> dec_fir_async/22(imag10)
  real24/1 -> dec_fir_async/49(real24)
  real16/1 -> dec_fir_async/33(real16)
  Constant27/1 -> dec_fir_async/52(imag25)
  real23/1 -> dec_fir_async/47(real23)
  Constant12/1 -> dec_fir_async/24(imag11)
  Constant33/1 -> dec_fir_async/64(imag31)
  real1/1 -> dec_fir_async/3(real1)
  Constant3/1 -> dec_fir_async/8(imag3)
  Constant28/1 -> dec_fir_async/54(imag26)
  dec_fir_async/3(dv_out) -> valid_out/1
  valid_in/1 -> dec_fir_async/2(dv_in)

== system decimation/conv_bus0/conv_ob0 ==
  i : Inport
  Concat : xbsIndex_r4/Concat  num_inputs=2  dbl_ovrd=off  block_type=concat
  Inverter : xbsIndex_r4/Inverter  en=off  latency=0  dbl_ovrd=off  block_type=inv
      settings: block_version=11.4
  Reinterpret : xbsIndex_r4/Reinterpret  force_arith_type=on  arith_type="Signed  (2's comp)"  force_bin_pt=on  bin_pt=7  block_type=reinterpret
      settings: infoedit="Changes signal type without altering the binary representation.   You can changed the signal between signed and unsigned, and relocate the binary point.<br><br>Hardware notes: In hardware this block costs nothing.<br><br>Example:  Suppose the input is 6 bits wide, signed, with 2 fractional bits, and the output is forced to unsigned with 0 fractional bits.  Then an input of -2.0 (1110.00 in binary 2's complement) becomes an output of 56 (111000 in binary)."
  Slice : xbsIndex_r4/Slice  nbits=1  boolean_output=off  mode=Upper Bit Location + Width  bit1=0  base1=MSB of Input  bit0=0  base0=LSB of Input  dbl_ovrd=off  block_type=slice
  Slice1 : xbsIndex_r4/Slice  nbits=7  boolean_output=off  mode=Upper Bit Location + Width  bit1=-1  base1=MSB of Input  bit0=0  base0=LSB of Input  dbl_ovrd=off  block_type=slice
  q : Outport
  wires:
  Reinterpret/1 -> q/1
  i/1 -> Slice1/1, Slice/1
  Concat/1 -> Reinterpret/1
  Slice1/1 -> Concat/2
  Inverter/1 -> Concat/1
  Slice/1 -> Inverter/1

== system decimation/conv_bus0/conv_ob1 ==
  i : Inport
  Concat : xbsIndex_r4/Concat  num_inputs=2  dbl_ovrd=off  block_type=concat
  Inverter : xbsIndex_r4/Inverter  en=off  latency=0  dbl_ovrd=off  block_type=inv
      settings: block_version=11.4
  Reinterpret : xbsIndex_r4/Reinterpret  force_arith_type=on  arith_type="Signed  (2's comp)"  force_bin_pt=on  bin_pt=7  block_type=reinterpret
      settings: infoedit="Changes signal type without altering the binary representation.   You can changed the signal between signed and unsigned, and relocate the binary point.<br><br>Hardware notes: In hardware this block costs nothing.<br><br>Example:  Suppose the input is 6 bits wide, signed, with 2 fractional bits, and the output is forced to unsigned with 0 fractional bits.  Then an input of -2.0 (1110.00 in binary 2's complement) becomes an output of 56 (111000 in binary)."
  Slice : xbsIndex_r4/Slice  nbits=1  boolean_output=off  mode=Upper Bit Location + Width  bit1=0  base1=MSB of Input  bit0=0  base0=LSB of Input  dbl_ovrd=off  block_type=slice
  Slice1 : xbsIndex_r4/Slice  nbits=7  boolean_output=off  mode=Upper Bit Location + Width  bit1=-1  base1=MSB of Input  bit0=0  base0=LSB of Input  dbl_ovrd=off  block_type=slice
  q : Outport
  wires:
  Slice/1 -> Inverter/1
  Inverter/1 -> Concat/1
  Slice1/1 -> Concat/2
  Concat/1 -> Reinterpret/1
  i/1 -> Slice/1, Slice1/1
  Reinterpret/1 -> q/1

== system decimation/conv_bus0/conv_ob10 ==
  i : Inport
  Concat : xbsIndex_r4/Concat  num_inputs=2  dbl_ovrd=off  block_type=concat
  Inverter : xbsIndex_r4/Inverter  en=off  latency=0  dbl_ovrd=off  block_type=inv
      settings: block_version=11.4
  Reinterpret : xbsIndex_r4/Reinterpret  force_arith_type=on  arith_type="Signed  (2's comp)"  force_bin_pt=on  bin_pt=7  block_type=reinterpret
      settings: infoedit="Changes signal type without altering the binary representation.   You can changed the signal between signed and unsigned, and relocate the binary point.<br><br>Hardware notes: In hardware this block costs nothing.<br><br>Example:  Suppose the input is 6 bits wide, signed, with 2 fractional bits, and the output is forced to unsigned with 0 fractional bits.  Then an input of -2.0 (1110.00 in binary 2's complement) becomes an output of 56 (111000 in binary)."
  Slice : xbsIndex_r4/Slice  nbits=1  boolean_output=off  mode=Upper Bit Location + Width  bit1=0  base1=MSB of Input  bit0=0  base0=LSB of Input  dbl_ovrd=off  block_type=slice
  Slice1 : xbsIndex_r4/Slice  nbits=7  boolean_output=off  mode=Upper Bit Location + Width  bit1=-1  base1=MSB of Input  bit0=0  base0=LSB of Input  dbl_ovrd=off  block_type=slice
  q : Outport
  wires:
  Slice/1 -> Inverter/1
  Inverter/1 -> Concat/1
  Slice1/1 -> Concat/2
  Concat/1 -> Reinterpret/1
  i/1 -> Slice/1, Slice1/1
  Reinterpret/1 -> q/1

== system decimation/conv_bus0/conv_ob11 ==
  i : Inport
  Concat : xbsIndex_r4/Concat  num_inputs=2  dbl_ovrd=off  block_type=concat
  Inverter : xbsIndex_r4/Inverter  en=off  latency=0  dbl_ovrd=off  block_type=inv
      settings: block_version=11.4
  Reinterpret : xbsIndex_r4/Reinterpret  force_arith_type=on  arith_type="Signed  (2's comp)"  force_bin_pt=on  bin_pt=7  block_type=reinterpret
      settings: infoedit="Changes signal type without altering the binary representation.   You can changed the signal between signed and unsigned, and relocate the binary point.<br><br>Hardware notes: In hardware this block costs nothing.<br><br>Example:  Suppose the input is 6 bits wide, signed, with 2 fractional bits, and the output is forced to unsigned with 0 fractional bits.  Then an input of -2.0 (1110.00 in binary 2's complement) becomes an output of 56 (111000 in binary)."
  Slice : xbsIndex_r4/Slice  nbits=1  boolean_output=off  mode=Upper Bit Location + Width  bit1=0  base1=MSB of Input  bit0=0  base0=LSB of Input  dbl_ovrd=off  block_type=slice
  Slice1 : xbsIndex_r4/Slice  nbits=7  boolean_output=off  mode=Upper Bit Location + Width  bit1=-1  base1=MSB of Input  bit0=0  base0=LSB of Input  dbl_ovrd=off  block_type=slice
  q : Outport
  wires:
  Reinterpret/1 -> q/1
  i/1 -> Slice1/1, Slice/1
  Concat/1 -> Reinterpret/1
  Slice1/1 -> Concat/2
  Inverter/1 -> Concat/1
  Slice/1 -> Inverter/1

== system decimation/conv_bus0/conv_ob12 ==
  i : Inport
  Concat : xbsIndex_r4/Concat  num_inputs=2  dbl_ovrd=off  block_type=concat
  Inverter : xbsIndex_r4/Inverter  en=off  latency=0  dbl_ovrd=off  block_type=inv
      settings: block_version=11.4
  Reinterpret : xbsIndex_r4/Reinterpret  force_arith_type=on  arith_type="Signed  (2's comp)"  force_bin_pt=on  bin_pt=7  block_type=reinterpret
      settings: infoedit="Changes signal type without altering the binary representation.   You can changed the signal between signed and unsigned, and relocate the binary point.<br><br>Hardware notes: In hardware this block costs nothing.<br><br>Example:  Suppose the input is 6 bits wide, signed, with 2 fractional bits, and the output is forced to unsigned with 0 fractional bits.  Then an input of -2.0 (1110.00 in binary 2's complement) becomes an output of 56 (111000 in binary)."
  Slice : xbsIndex_r4/Slice  nbits=1  boolean_output=off  mode=Upper Bit Location + Width  bit1=0  base1=MSB of Input  bit0=0  base0=LSB of Input  dbl_ovrd=off  block_type=slice
  Slice1 : xbsIndex_r4/Slice  nbits=7  boolean_output=off  mode=Upper Bit Location + Width  bit1=-1  base1=MSB of Input  bit0=0  base0=LSB of Input  dbl_ovrd=off  block_type=slice
  q : Outport
  wires:
  Slice/1 -> Inverter/1
  Inverter/1 -> Concat/1
  Slice1/1 -> Concat/2
  Concat/1 -> Reinterpret/1
  i/1 -> Slice/1, Slice1/1
  Reinterpret/1 -> q/1

== system decimation/conv_bus0/conv_ob13 ==
  i : Inport
  Concat : xbsIndex_r4/Concat  num_inputs=2  dbl_ovrd=off  block_type=concat
  Inverter : xbsIndex_r4/Inverter  en=off  latency=0  dbl_ovrd=off  block_type=inv
      settings: block_version=11.4
  Reinterpret : xbsIndex_r4/Reinterpret  force_arith_type=on  arith_type="Signed  (2's comp)"  force_bin_pt=on  bin_pt=7  block_type=reinterpret
      settings: infoedit="Changes signal type without altering the binary representation.   You can changed the signal between signed and unsigned, and relocate the binary point.<br><br>Hardware notes: In hardware this block costs nothing.<br><br>Example:  Suppose the input is 6 bits wide, signed, with 2 fractional bits, and the output is forced to unsigned with 0 fractional bits.  Then an input of -2.0 (1110.00 in binary 2's complement) becomes an output of 56 (111000 in binary)."
  Slice : xbsIndex_r4/Slice  nbits=1  boolean_output=off  mode=Upper Bit Location + Width  bit1=0  base1=MSB of Input  bit0=0  base0=LSB of Input  dbl_ovrd=off  block_type=slice
  Slice1 : xbsIndex_r4/Slice  nbits=7  boolean_output=off  mode=Upper Bit Location + Width  bit1=-1  base1=MSB of Input  bit0=0  base0=LSB of Input  dbl_ovrd=off  block_type=slice
  q : Outport
  wires:
  Reinterpret/1 -> q/1
  i/1 -> Slice1/1, Slice/1
  Concat/1 -> Reinterpret/1
  Slice1/1 -> Concat/2
  Inverter/1 -> Concat/1
  Slice/1 -> Inverter/1

== system decimation/conv_bus0/conv_ob14 ==
  i : Inport
  Concat : xbsIndex_r4/Concat  num_inputs=2  dbl_ovrd=off  block_type=concat
  Inverter : xbsIndex_r4/Inverter  en=off  latency=0  dbl_ovrd=off  block_type=inv
      settings: block_version=11.4
  Reinterpret : xbsIndex_r4/Reinterpret  force_arith_type=on  arith_type="Signed  (2's comp)"  force_bin_pt=on  bin_pt=7  block_type=reinterpret
      settings: infoedit="Changes signal type without altering the binary representation.   You can changed the signal between signed and unsigned, and relocate the binary point.<br><br>Hardware notes: In hardware this block costs nothing.<br><br>Example:  Suppose the input is 6 bits wide, signed, with 2 fractional bits, and the output is forced to unsigned with 0 fractional bits.  Then an input of -2.0 (1110.00 in binary 2's complement) becomes an output of 56 (111000 in binary)."
  Slice : xbsIndex_r4/Slice  nbits=1  boolean_output=off  mode=Upper Bit Location + Width  bit1=0  base1=MSB of Input  bit0=0  base0=LSB of Input  dbl_ovrd=off  block_type=slice
  Slice1 : xbsIndex_r4/Slice  nbits=7  boolean_output=off  mode=Upper Bit Location + Width  bit1=-1  base1=MSB of Input  bit0=0  base0=LSB of Input  dbl_ovrd=off  block_type=slice
  q : Outport
  wires:
  Reinterpret/1 -> q/1
  i/1 -> Slice1/1, Slice/1
  Concat/1 -> Reinterpret/1
  Slice1/1 -> Concat/2
  Inverter/1 -> Concat/1
  Slice/1 -> Inverter/1
